simulink model "Simulink_Sem_Restricao"  (Simulink 8.2)
settings: Solver=ode4  SolverMode=SingleTasking  StartTime=0.0  StopTime=500  FixedStep=0.01  RelTol=1e-3
InitFcn:
  | Main_Simulink_Sem_Restricao;
values from neighbouring files (symbols this model uses):
  A1 = [   1   0.1 ... (first row only)    [MatrizesEspacoEstados.m]
  B1 = [0 ... (first row only)    [MatrizesEspacoEstados.m]
  C = eye(n)    [MatrizesEspacoEstados.m]
  D = 0*C(:,n)    [MatrizesEspacoEstados.m]
  T = 1    [VariaveisDiversas_Restricoes.m]
  xk0 = [80; 0.4]    [xk_0.m]
undefined symbols (not defined in the file): A, B
settings Model: Creator=Kawakami  LastModifiedBy=Eduardo
settings DataIOCC: LimitDataPoints=off  SaveOutput=off  SaveTime=off  TimeSaveName=t  SignalLoggingName=sigsOut
settings OptimizationCC: BooleanDataType=off
settings DebuggingCC: SaveWithParameterizedLinksMsg=none  SignalResolutionControl=TryResolveAllWithWarning  SolverPrmCheckMsg=none  MultiTaskDSMMsg=warning  MultiTaskCondExecSysMsg=none
settings HardwareCC: TargetUnknown=on
settings RTWCC: IncludeERTFirstTime=on

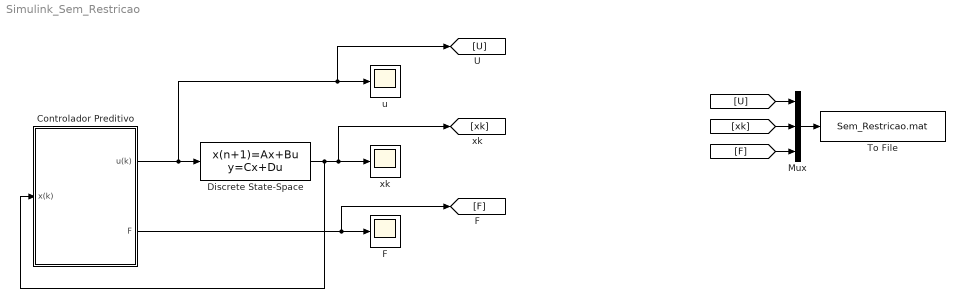
== system Simulink_Sem_Restricao ==
  "Controlador Preditivo  " : Subsystem  mask{A=A, B=B, T=T}
      mask prompts: A "Matriz Agregada A"; B "Matriz Agregada B"; T "T (passo da simulação)"
  Discrete State-Space : DiscreteStateSpace  A=A1  B=B1  C=C  D=D  X0=xk0
  F : Scope
      settings: YMin=-1.25  YMax=2.25  SaveName=ScopeData2
  Mux : Mux  Inputs=3
  To File : ToFile  Filename=Sem_Restricao.mat  MatrixName=SemRestricao
  u : Scope
      settings: TimeRange=10  YMin=-2  YMax=0.5
  xk : Scope
      settings: YMin=-1.25  YMax=2.25
  wires:
  "Controlador Preditivo  "/1(u(k)) -> [U], u/1, Discrete State-Space/1
  Discrete State-Space/1 -> xk/1, [xk], "Controlador Preditivo  "/1(x(k))
  "Controlador Preditivo  "/2(F) -> [F], F/1
  Mux/1 -> To File/1
  [F] -> Mux/3
  [xk] -> Mux/2
  [U] -> Mux/1

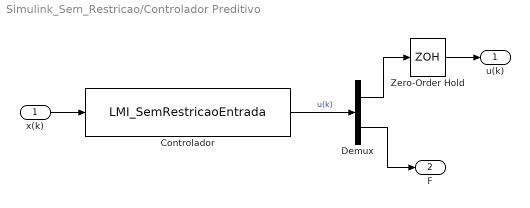
== system Simulink_Sem_Restricao/Controlador Preditivo   ==
  x(k) : Inport
  Controlador : S-Function  FunctionName=LMI_SemRestricaoEntrada  Parameters=A, B, T  EnableBusSupport=off
  Demux : Demux  Outputs=2
  Zero-Order Hold : ZeroOrderHold  SampleTime=T
  u(k) : Outport
  F : Outport  Port=2
  wires:
  Zero-Order Hold/1 -> u(k)/1
  x(k)/1 -> Controlador/1
  Controlador/1 -> Demux/1  "u(k)"
  Demux/1 -> Zero-Order Hold/1
  Demux/2 -> F/1
